simulink model "SinglePulseModel_n_4"  (R2014a)
settings: Solver=FixedStepDiscrete  StartTime=0.0  StopTime=200  RelTol=1e-3
InitFcn:
  | initialization_n_20;
StopFcn:
  | OutputPlotting;
values from neighbouring files (symbols this model uses):
  delays = tim(T,n,1:n)    [initialization.m]    (also in initialization_n_20.m; initialization_n_6.m; initialization_new.m = [10e-9, 14.33e-9, 18.66e-9]; initialization_pulsePicking.m = [])
libraries: BlockLib x15, dspsrcs4 x1
settings Model: Creator=kunalmenda  LastModifiedBy=Alexander
settings DebuggingCC: MergeDetectMultiDrivingBlocksExec=error

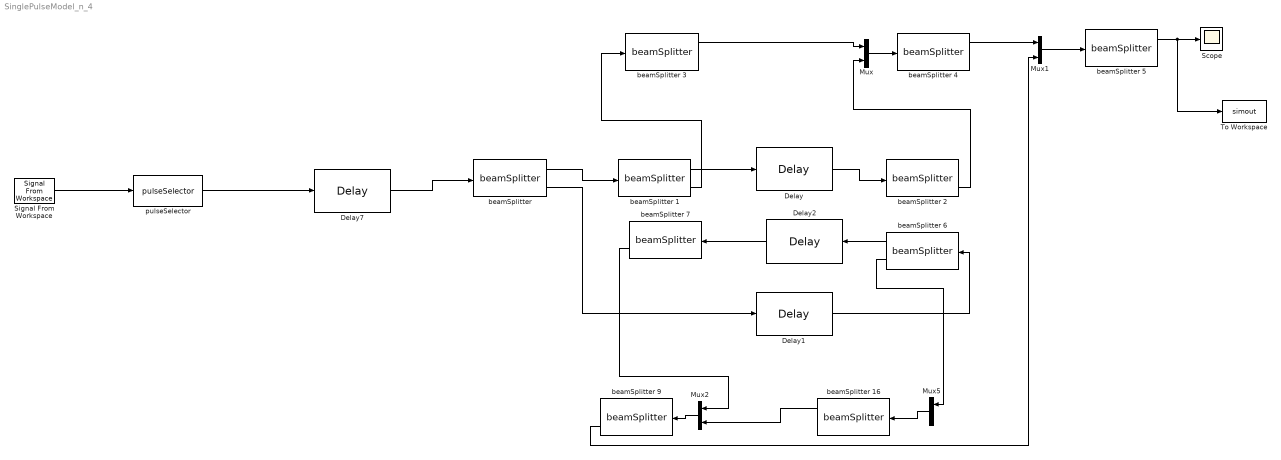
== system SinglePulseModel_n_4 ==
  Delay : BlockLib/Delay  DelayAmt=delays(2)-delays(1)
  Delay1 : BlockLib/Delay  DelayAmt=delays(3)-delays(1)
  Delay2 : BlockLib/Delay  DelayAmt=delays(2)-delays(1)
  Delay7 : BlockLib/Delay  DelayAmt=delays(1)
  Mux{,1..2,5} (4 alike) : Mux  Inputs=2
  Scope : Scope
  Signal From Workspace : dspsrcs4/Signal From Workspace  X=inputsignal  Ts=1  nsamps=1  OutputAfterFinalValue=Setting to zero  ignoreOrWarnInputAndFrameLengths=off
  To Workspace : ToWorkspace  VariableName=simout  SaveFormat=Timeseries  SampleTime=-1
  beamSplitter {,1..7,9,16} (10 alike) : BlockLib/beamSplitter 
  pulseSelector : BlockLib/pulseSelector  OutputDimensions=1  PCID=1
  wires:
  "beamSplitter "/1 -> beamSplitter 1/1
  beamSplitter 2/2 -> Mux/2
  beamSplitter 3/1 -> Mux/1
  Mux/1 -> beamSplitter 4/1
  Mux1/1 -> beamSplitter 5/1
  Delay/1 -> beamSplitter 2/1
  beamSplitter 1/2 -> beamSplitter 3/1
  Delay2/1 -> beamSplitter 7/1
  beamSplitter 7/2 -> Mux2/1
  Mux2/1 -> beamSplitter 9/1
  beamSplitter 5/1 -> To Workspace/1, Scope/1
  "beamSplitter "/2 -> Delay1/1
  beamSplitter 1/1 -> Delay/1
  Mux5/1 -> beamSplitter 16/1
  beamSplitter 6/2 -> Mux5/1
  beamSplitter 16/1 -> Mux2/2
  Delay7/1 -> "beamSplitter "/1
  beamSplitter 6/1 -> Delay2/1
  pulseSelector/1 -> Delay7/1
  Signal From Workspace/1 -> pulseSelector/1
  Delay1/1 -> beamSplitter 6/1
  beamSplitter 4/1 -> Mux1/1
  beamSplitter 9/2 -> Mux1/2
